simulink model "AUAV_V3_TestSensors"  (R2015a)
settings: Solver=FixedStepDiscrete  StartTime=0.0  StopTime=10.0  FixedStep=T  RelTol=1e-3
PreLoadFcn:
  | %T = 0.0025;
  | MavlinkBus;
  | mcuInit;
  | % Baro Altitude Computation
  | % =========================
  | basePressure = 98192.64;
  | baseTemp = 288.215;
  | lapseRate = -0.00198122;
  | baseHeight = 0;
values from neighbouring files (symbols this model uses):
  apSampleTime = 0.01    [mcuInit.m]
  latlong_WP = 1    [mcuInit.m]
  mavlink_attitude_t = Simulink.Bus    [MavlinkBusMarcello.m]
  mavlink_gps_raw_int_t = Simulink.Bus    [MavlinkBus.m]    (also in MavlinkBusMarcello.m)
  mavlink_raw_imu_t = Simulink.Bus    [MavlinkBus.m]    (also in MavlinkBusMarcello.m)
  mavlink_scaled_pressure_t = Simulink.Bus    [MavlinkBus.m]    (also in MavlinkBusMarcello.m)
  mavlink_servo_output_raw_t = Simulink.Bus    [MavlinkBusMarcello.m]
  mavlink_slugs_navigation_t = Simulink.Bus    [MavlinkBusMarcello.m]
  mavlink_sys_status_t = Simulink.Bus    [MavlinkBus.m]    (also in MavlinkBusMarcello.m)
  T = 0.01    [mcuInit.m]
  Xpoints = [0 0]    [mcuInit.m]
  Ypoints = [0 0]    [mcuInit.m]
  Zpoints = [0 0]    [mcuInit.m]
undefined symbols (not defined in the file or in its folder): A0, A14, A15, A2, A3, A4, A5, A6, accBiasRateLimit, B0, bankCommandLimit, barAdjust, baroCutoff, baroCutTemp, cubeAccelGain16405, cubeGyroGain16405, cubeMagGain16405, D0, D11, D7, D8, daLimit, data, daTrimMax, daTrimMin, deLimit, deTrimMax, deTrimMin, drLimit, drTrimMax, drTrimMin, dtLimit, dtTrimMax, dtTrimMin, F2, F3, G0, G13, G15, gaind, GS_location, gyroBiasRateLimit, IC1max, IPStar, ISA_g, Max, maxAcc, MaxDwnPthStar, maxDynPressure, maxEta, mlParamInterface, ms, OC1max, P112, P125, P127, P16, P20, P21, P30 ... (+26)
undefined symbols (not defined in the file): baroOffset, baroScale, barTGain1, barTGain2, barTMean1, barTMean2, bda, bde, bdr, bdt, bICda, bICde, bICdr, bICdt, derivativesConstant, lowRateSensorCutoff, mainSensorCutoff, mda, mde, mdr, mdt, mICda, mICde, mICdr, mICdt, pitotOffset, pitotScale, pitTGain1, pitTGain2, pitTMean1, pitTMean2, powerOffset, powerScale, pressureSensorCutoff, tempOffset, tempScale, vzCutoff, xCutoff, yCutoff
libraries: MCHP_Blockset x158, simulink x84, SLUGS_Library x31, aerolibconvert2 x6, aerolibutil x4, aerolibtransform2 x3, dspmtrx3 x2, aerolibobsolete x2
(part 9 of 24)

== system AUAV_V3_TestSensors/Inner Loop// Navigation/Longitudinal Channel Encaps [updated 4.28.16] ==
  U_c : Inport
  dyn P : Inport  Port=2
  U_hold PID Gains : Inport  Port=3
  dT_trim : Inport  Port=4
  h_c : Inport  Port=5
  h_m : Inport  Port=6
  he2th PI Gains : Inport  Port=7
  Roll to Height FF : Inport  Port=8
  theta_m : Inport  Port=9
  th2dE PID Gains : Inport  Port=10
  dE_trim : Inport  Port=11
  Manual? : Inport  Port=12
  phi_m : Inport  Port=13
  dt FF Gain : Inport  Port=14
  Constant3 : Constant  Value=[100 100 100]  OutDataTypeStr=single
  Longitudinal Channel : Subsystem  AncestorBlock=SLUGS_Library/Control Blocks/Longitudinal Channel
  mlNavigation : DataStoreWrite  DialogController=Simulink.DDGSource  DataStoreName=mlNavigation  DataStoreElements=mlNavigation.u_m#mlNavigation.theta_c#mlNavigation.h_c
  dE : Outport
  dT : Outport  Port=2
  theta_C : Outport  Port=3
  h_c_in : Outport  Port=4
  U_m : Outport  Port=5
  wires:
  U_c/1 -> Longitudinal Channel/1(U_c)
  dyn P/1 -> Longitudinal Channel/2(dyn P)
  U_hold PID Gains/1 -> Longitudinal Channel/3(U_hold PID Gains)
  dT_trim/1 -> Longitudinal Channel/4(dT_trim)
  h_m/1 -> Longitudinal Channel/6(h_m)
  theta_m/1 -> Longitudinal Channel/9(theta_m)
  dE_trim/1 -> Longitudinal Channel/11(dE_trim)
  Manual?/1 -> Longitudinal Channel/12(Manual?)
  he2th PI Gains/1 -> Longitudinal Channel/7(he2th PI Gains)
  Roll to Height FF/1 -> Longitudinal Channel/8(Roll to Height FF)
  th2dE PID Gains/1 -> Longitudinal Channel/10(th2dE PID Gains)
  dt FF Gain/1 -> Longitudinal Channel/14(dt FF Gain)
  h_c/1 -> Longitudinal Channel/5(h_c)
  phi_m/1 -> Longitudinal Channel/13(phi_m)
  Longitudinal Channel/1(dE) -> dE/1  "U"
  Longitudinal Channel/2(dT) -> dT/1
  Longitudinal Channel/3(h_c_in) -> mlNavigation/3, h_c_in/1
  Longitudinal Channel/4(U_m) -> mlNavigation/1, U_m/1
  Longitudinal Channel/5(theta_C) -> mlNavigation/2, theta_C/1
  Constant3/1 -> Longitudinal Channel/15(GS Location)

== system AUAV_V3_TestSensors/Inner Loop// Navigation/Navigation Encaps [updated 4.28.16] ==
  Puav : Inport  SampleTime=apSampleTime
  Max WP Idx : Inport  Port=2
  Vxyz : Inport  Port=3  SampleTime=apSampleTime
  T*(m) : Inport  Port=4
  U_c : Inport  Port=5
  WPFly : Inport  Port=6
  TurnLeadTime : Inport  Port=7
  RTB : Inport  Port=8
  Mobile Location : Inport  Port=9
  Follow Mobile? : Inport  Port=10
  MidLvl h_c : Inport  Port=11
  isApManual? : Inport  Port=12
  ISR Scale : Inport  Port=13
  Data Type Conversion : DataTypeConversion  OutDataTypeStr=uint8
  Get ISR Location : DataStoreRead  DialogController=Simulink.DDGSource  DataStoreName=mlISR  DataStoreElements=mlISR.latitude#mlISR.longitude#mlISR.height
  Get Nav Mode : DataStoreRead  DialogController=Simulink.DDGSource  DataStoreName=mlHeartbeatLocal  DataStoreElements=mlHeartbeatLocal.custom_mode
  Mux : Mux  Inputs=3
  Navigation : Subsystem  AncestorBlock=SLUGS_Library/Navigation/Navigation
  h_c : Outport
  phi_c : Outport  Port=2
  ISR Loc : Outport  Port=3
  "Puav " : Outport  Port=4
  wires:
  T*(m)/1 -> Navigation/2(T*(m))
  WPFly/1 -> Navigation/3(WPFly)
  RTB/1 -> Navigation/4(RTB)
  isApManual?/1 -> Navigation/5(isApManual?)
  Navigation/1(h_c) -> h_c/1
  Navigation/2(phi_c) -> phi_c/1
  Puav/1 -> Navigation/6(Puav)
  Navigation/4("Puav ") -> "Puav "/1
  Max WP Idx/1 -> Navigation/8(Max WP Idx)
  Vxyz/1 -> Navigation/9(Vxyz)
  U_c/1 -> Navigation/10(U_c)
  TurnLeadTime/1 -> Navigation/11(TurnLeadTime)
  Mobile Location/1 -> Navigation/12(Mobile Location)
  Follow Mobile?/1 -> Navigation/13(Follow Mobile?)
  MidLvl h_c/1 -> Navigation/14(MidLvl h_c)
  ISR Scale/1 -> Navigation/15(ISR Scale)
  Navigation/3(ISR Loc) -> ISR Loc/1
  Mux/1 -> Navigation/7(ISR Location)
  Get ISR Location/2 -> Mux/2
  Get ISR Location/1 -> Mux/1
  Get ISR Location/3 -> Mux/3
  Get Nav Mode/1 -> Data Type Conversion/1
  Data Type Conversion/1 -> Navigation/1(NavMode)

== system AUAV_V3_TestSensors/Inner Loop// Navigation/Protect NaNs ==
  In1 : Inport
  Integer Delay3 : Delay  DelayLength=1  InputProcessing=Inherited  SampleTime=T
  Relational Operator2 : RelationalOperator  Operator===  OutDataTypeStr=uint(8)
  Switch3 : Switch  Criteria=u2 > Threshold  Threshold=0.3  SampleTime=.01
  Out1 : Outport
  wires:
  Integer Delay3/1 -> Switch3/3
  Switch3/1 -> Out1/1, Integer Delay3/1
  In1/1 -> Relational Operator2/2, Relational Operator2/1, Switch3/1
  Relational Operator2/1 -> Switch3/2

== system AUAV_V3_TestSensors/Position_and_Attitude_Filter/Attitude Complimentary Filter COG ==
  A_sens : Inport  PortDimensions=3
  XY Orient : Inport  Port=2  OutDataTypeStr=single
  Gyros : Inport  Port=3  PortDimensions=3
  Vxyd_hat : Inport  Port=4  PortDimensions=3
  acc_bias : Inport  Port=5  PortDimensions=3
  3D Filter : Subsystem  AncestorBlock=SLUGS_Library/Singnal Routing & Conditioning/3D Filter  RTWFcnName=TustinFilter3D  mask{zval=[], pval=[0], kval=1, TSample=0.01}
      mask prompts: zval "Zeros"; pval "Poles"; kval "Gains"; TSample "Sample Time"
      settings: RTWFcnNameOpts=User specified  RTWFileNameOpts=Use function name
      mask Display:
      | droots(zval,pval,kval)
      | port_label('input',1,'3D')
  3x3 Cross Product : aerolibutil/3x3 Cross Product
  3x3 Cross Product1 : aerolibutil/3x3 Cross Product
  3x3 Cross Product2 : aerolibutil/3x3 Cross Product
  Add : Sum  Inputs=++--
  Bias Rate Limiter : RateLimiter  RisingSlewLimit=gyroBiasRateLimit  FallingSlewLimit=-gyroBiasRateLimit  SampleTimeMode=inherited
  Constant1 : Constant  Value=0  OutDataTypeStr=single
  Data Type Conversion : DataTypeConversion  OutDataTypeStr=single
  Demux : Demux  Outputs=3
  Demux1 : Demux  Outputs=3
  "Deriv " : Subsystem
  Direction Cosine Matrix to Rotation Angles : aerolibtransform2/Direction Cosine Matrix to Rotation Angles  rotationOrder=ZYX  lim=Default
      settings: AttributesFormatString=Rotation Order: %<rotationOrder>
  Discrete-Time Integrator1 : DiscreteIntegrator  InitialCondition=q_quat  SampleTime=apSampleTime  LimitOutput=on  UpperSaturationLimit=[1 1 1 1]  LowerSaturationLimit=[-1 -1 -1 -1]
  Embedded MATLAB Function : MATLAB Function  TreatAsAtomicUnit=on
  Gain : Gain  Gain=0.1
  Gain1 : Gain  Gain=30
  Integer Delay : Delay  DelayLength=1  InputProcessing=Inherited
  Mux : Mux  Inputs=3
  Normalize Vector1 : Subsystem  AncestorBlock=SLUGS_Library/Navigation/Normalize Vector
  Normalize Vector2 : Subsystem  AncestorBlock=SLUGS_Library/Navigation/Normalize Vector
  Product1 : Product  Multiplication=Matrix(*)  RndMeth=Zero
  Product2 : Product  Multiplication=Matrix(*)  RndMeth=Zero
  Quaternion Normalize : aerolibutil/Quaternion Normalize
  Quaternions to Direction Cosine Matrix : aerolibtransform2/Quaternions to  Direction Cosine Matrix
  Submatrix : dspmtrx3/Submatrix  RowSpan=Range of rows  RowStartMode=First  RowStartIndex=1  RowEndMode=Last  RowEndIndex=1  ColSpan=One column  ColStartMode=Last  ColStartIndex=1  ColEndMode=Last  ColEndIndex=1
  Submatrix1 : dspmtrx3/Submatrix  RowSpan=One row  RowStartMode=First  RowStartIndex=1  RowEndMode=Last  RowEndIndex=1  ColSpan=All columns  ColStartMode=Last  ColStartIndex=1  ColEndMode=Last  ColEndIndex=1
  Sum1 : Sum  Inputs=++|
  Sum3 : Sum  Inputs=++|
  Sum4 : Sum  Inputs=++|
  myMux Fun2 : MATLAB Function  TreatAsAtomicUnit=on
  q dot calc : MATLAB Function  TreatAsAtomicUnit=on
  euler_hat : Outport
  pqr_hat : Outport  Port=2
  Gyro Bias : Outport  Port=3
  RL2B : Outport  Port=4
  wires:
  Bias Rate Limiter/1 -> Gyro Bias/1, Sum3/2
  Product2/1 -> Gain1/1
  Gain1/1 -> Sum4/1
  Normalize Vector2/1(Normalized) -> 3x3 Cross Product2/1
  myMux Fun2/1(y) -> Normalize Vector2/1(Vector)
  Constant1/1 -> myMux Fun2/3(u3)
  Demux1/2 -> myMux Fun2/2(u2)
  Demux1/1 -> myMux Fun2/1(u1)
  Submatrix1/1 -> Demux1/1
  Sum1/1 -> q dot calc/2(om_hat), Integer Delay/1  "om_hat"
  q dot calc/1(q_dot) -> Discrete-Time Integrator1/1
  Submatrix/1 -> 3x3 Cross Product/2  "g_hat"
  Sum4/1 -> Gain/1, 3D Filter/1(In1)
  3x3 Cross Product1/1 -> Add/1
  A_sens/1 -> Add/3
  Normalize Vector1/1(Normalized) -> 3x3 Cross Product/1
  3x3 Cross Product/1 -> Sum4/2
  Quaternions to Direction Cosine Matrix/1 -> Submatrix1/1, Product2/1, Product1/1, Submatrix/1, RL2B/1, Direction Cosine Matrix to Rotation Angles/1  "RLT2B"
  Integer Delay/1 -> 3x3 Cross Product1/1
  Discrete-Time Integrator1/1 -> Quaternion Normalize/1  "q1"
  Quaternion Normalize/1 -> Quaternions to Direction Cosine Matrix/1, q dot calc/1(q)
  "Deriv "/1(ydot) -> Add/2
  Add/1 -> Normalize Vector1/1(Vector)
  acc_bias/1 -> Add/4
  Product1/1 -> 3x3 Cross Product1/2, "Deriv "/1(y)
  Vxyd_hat/1 -> Product1/2
  3D Filter/1(Out1) -> Bias Rate Limiter/1
  Gyros/1 -> Sum3/1
  Gain/1 -> Sum1/2
  Sum3/1 -> Sum1/1, pqr_hat/1  "Gyro Err"
  XY Orient/1 -> 3x3 Cross Product2/2
  3x3 Cross Product2/1 -> Product2/2
  Demux/1 -> Embedded MATLAB Function/1(u)
  Mux/1 -> euler_hat/1
  Embedded MATLAB Function/1(y) -> Mux/3
  Direction Cosine Matrix to Rotation Angles/1 -> Data Type Conversion/1
  Demux/2 -> Mux/2
  Demux/3 -> Mux/1
  Data Type Conversion/1 -> Demux/1

== system AUAV_V3_TestSensors/Position_and_Attitude_Filter/COG.SOG2V ==
  COG_D : Inport
  SOG : Inport  Port=2
  Angle Conversion : aerolibconvert2/Angle Conversion  IU=deg  OU=rad
  Constant : Constant  Value=0  OutDataTypeStr=single
  Product : Product  RndMeth=Zero
  Product1 : Product  RndMeth=Zero
  Subsystem5 : Subsystem  AncestorBlock=SLUGS_Library/Subsystem5
  myMux Fun2 : MATLAB Function  TreatAsAtomicUnit=on
  Vnorth : Outport
  Veast : Outport  Port=2
  XY Orient : Outport  Port=3
  wires:
  Product1/1 -> Vnorth/1
  Product/1 -> Veast/1
  SOG/1 -> Product1/1, Product/2
  Angle Conversion/1 -> Subsystem5/1(u)
  Subsystem5/1(sin(u)) -> Product/1, myMux Fun2/2(u2)
  Subsystem5/2(cos(u)) -> Product1/2, myMux Fun2/1(u1)
  COG_D/1 -> Angle Conversion/1
  Constant/1 -> myMux Fun2/3(u3)
  myMux Fun2/1(y) -> XY Orient/1

== system AUAV_V3_TestSensors/Position_and_Attitude_Filter/Compute GS Location ==
  GS Location : Inport
  Demux : Demux  Outputs=3
  Geod2ECEF1 : Subsystem  mask{Re=6378137, Rp=6356752.3142}
      mask prompts: Re "Enter equatorial radius, m"; Rp "Enter polar radius,m"
  Mux1 : Mux  Inputs=2
  Mux2 : Mux  Inputs=3
  "Lat, Lon" : Outport
  R_in : Outport  Port=2
  wires:
  Geod2ECEF1/3("Ze, m ") -> Mux2/3
  Geod2ECEF1/1("Xe, m ") -> Mux2/1
  Geod2ECEF1/2("Ye, m ") -> Mux2/2
  Demux/1 -> Geod2ECEF1/1("height, m")
  Demux/2 -> Mux1/2, Geod2ECEF1/2("lat, deg")
  Demux/3 -> Mux1/1, Geod2ECEF1/3(lon,deg)
  GS Location/1 -> Demux/1
  Mux1/1 -> "Lat, Lon"/1
  Mux2/1 -> R_in/1  "R_in"

== system AUAV_V3_TestSensors/Position_and_Attitude_Filter/Enabled Subsystem ==
  In1 : Inport
  In2 : Inport  Port=2
  In3 : Inport  Port=3
  Enable : EnablePort
  Out1 : Outport
  Out2 : Outport  Port=2
  Out3 : Outport  Port=3
  wires:
  In1/1 -> Out1/1
  In2/1 -> Out2/1
  In3/1 -> Out3/1

== system AUAV_V3_TestSensors/Position_and_Attitude_Filter/GPS Update ==
  XYZ : Inport
  Data Type Conversion2 : DataTypeConversion  OutDataTypeStr=uint8
  Demux : Demux  Outputs=3
  Detect Change : Subsystem
  Detect Change1 : Subsystem
  Detect Change2 : Subsystem
  Rate Transition : RateTransition  OutPortSampleTime=T
  Saturation1 : Saturate  UpperLimit=1  LowerLimit=0  SampleTime=T
  Sum : Sum  Inputs=3
  Update? : Outport
  wires:
  Demux/1 -> Detect Change/1(Data)
  Demux/2 -> Detect Change1/1(Data)
  Demux/3 -> Detect Change2/1(Data)
  Detect Change/1(change?) -> Sum/1
  Detect Change1/1(change?) -> Sum/2
  Detect Change2/1(change?) -> Sum/3
  Sum/1 -> Saturation1/1
  XYZ/1 -> Rate Transition/1
  Saturation1/1 -> Data Type Conversion2/1
  Rate Transition/1 -> Demux/1
  Data Type Conversion2/1 -> Update?/1

== system AUAV_V3_TestSensors/Position_and_Attitude_Filter/Geod2LTP1 ==
  GS Lat,Lon : Inport
  GS ECEF : Inport  Port=2
  "Lat, deg(GPS)" : Inport  Port=3
  "Lon, deg(GPS)" : Inport  Port=4
  Hight,m(GPS) : Inport  Port=5
  ECEF2LTP (UEN) : Subsystem
      mask Display: plot(0,0,100,100,[45,40,35,40,40],[85,95,85,95,40],[85,95,85,95,40],[35,40,45,40,40],[60,40,10,20,10,14],[70,40,10,13,10,20],[56,45],[70,70],[60,60],[50,60],[60,60],[30,40],[50,60],[20,20],[30,40],[20,20],[45,55],[35,25],[75,65],[35,25])
  Geod2ECEF1 : Subsystem  mask{Re=6378137, Rp=6356752.3142}
      mask prompts: Re "Enter equatorial radius, m"; Rp "Enter polar radius,m"
  Mux : Mux  Inputs=3
  Reshape : Reshape  OutputDimensionality=Column vector (2-D)
  Reshape1 : Reshape
  Sum1 : Sum  Inputs=|+-  OutDataTypeStr=single  SaturateOnIntegerOverflow=on
  UEN 2 NEU : Gain  Gain=[0 0 1;0 1 0;1 0 0]  Multiplication=Matrix(K*u)  OutDataTypeStr=float('single')  SaturateOnIntegerOverflow=on  ParamDataTypeStr=Inherit: Same as input
  "NEU, m" : Outport
  wires:
  Reshape1/1 -> "NEU, m"/1
  Reshape/1 -> UEN 2 NEU/1
  Sum1/1 -> ECEF2LTP (UEN)/1(ECEF coordinates)
  Mux/1 -> Sum1/1  "r_mov"
  Hight,m(GPS)/1 -> Geod2ECEF1/1("height, m")
  ECEF2LTP (UEN)/1(Out) -> Reshape/1  "Moving Side"
  GS ECEF/1 -> Sum1/2
  GS Lat,Lon/1 -> ECEF2LTP (UEN)/2("Long, Lat")
  "Lon, deg(GPS)"/1 -> Geod2ECEF1/3(lon,deg)
  "Lat, deg(GPS)"/1 -> Geod2ECEF1/2("lat, deg")
  Geod2ECEF1/2("Ye, m ") -> Mux/2
  Geod2ECEF1/1("Xe, m ") -> Mux/1
  Geod2ECEF1/3("Ze, m ") -> Mux/3
  UEN 2 NEU/1 -> Reshape1/1

== system AUAV_V3_TestSensors/Position_and_Attitude_Filter/Position Filter ==
  NewGPS : Inport
  Baro Alt : Inport  Port=2
  RLT2B : Inport  Port=3
  GPS_XYD : Inport  Port=4
  Vnorth : Inport  Port=5
  Veast : Inport  Port=6
  SOG : Inport  Port=7
  A_sens(m/s^2) : Inport  Port=8
  Base Height (m) : Inport  Port=9
  BlendPosVel : Subsystem
  Vxyd_hat : Outport
  Pxyd_hat : Outport  Port=2
  acc_bias : Outport  Port=3
  wires:
  BlendPosVel/3(acc_bias) -> acc_bias/1
  BlendPosVel/1(Vxyd_hat) -> Vxyd_hat/1
  BlendPosVel/2(Pxyd_hat) -> Pxyd_hat/1
  Baro Alt/1 -> BlendPosVel/4(BaroAlt)
  Veast/1 -> BlendPosVel/3(Veast)
  Vnorth/1 -> BlendPosVel/2(Vnorth)
  NewGPS/1 -> BlendPosVel/6(NewGPS)
  RLT2B/1 -> BlendPosVel/5(RLT2B)
  GPS_XYD/1 -> BlendPosVel/1(GPS_NED)
  SOG/1 -> BlendPosVel/7(SOG)
  A_sens(m/s^2)/1 -> BlendPosVel/8(A_sens(m/s^2))
  Base Height (m)/1 -> BlendPosVel/9(Base Height)

== system AUAV_V3_TestSensors/RC_Driver/Mixing ==
  note: Pitch positif : go down
      | Yaw positive : turn left
  Pitch : Inport
  Roll : Inport  Port=2
  Sum : Sum  Inputs=-+  SaturateOnIntegerOverflow=on  OutDataTypeStr=Inherit: Same as first input
  Sum1 : Sum  SaturateOnIntegerOverflow=on  OutDataTypeStr=Inherit: Same as first input
  Cmd Servo Left : Outport
  Cmd Servo Right : Outport  Port=2
  wires:
  Pitch/1 -> Sum1/1, Sum/1
  Roll/1 -> Sum/2, Sum1/2
  Sum/1 -> Cmd Servo Left/1
  Sum1/1 -> Cmd Servo Right/1

== system AUAV_V3_TestSensors/Sensor_Data_Adapter/Initialize GS Location ==
  Enable : EnablePort
  Constant : Constant  Value=0
  Data Store Read1 : DataStoreRead  DataStoreName=mlGpsData  DataStoreElements=mlGpsData.lat#mlGpsData.lon#mlGpsData.alt
  Data Store Write : DataStoreWrite  DataStoreName=GS_INIT_FLAG
  Data Store Write1 : DataStoreWrite  DialogController=Simulink.DDGSource  DataStoreName=mlGSLocationFloat  DataStoreElements=mlGSLocationFloat.lat#mlGSLocationFloat.lon#mlGSLocationFloat.alt
  Data Type Conversion : DataTypeConversion
  Data Type Conversion1 : DataTypeConversion
  Data Type Conversion2 : DataTypeConversion
  wires:
  Data Store Read1/1 -> Data Type Conversion/1
  Data Store Read1/2 -> Data Type Conversion1/1
  Constant/1 -> Data Store Write/1
  Data Store Read1/3 -> Data Type Conversion2/1
  Data Type Conversion/1 -> Data Store Write1/1
  Data Type Conversion1/1 -> Data Store Write1/2
  Data Type Conversion2/1 -> Data Store Write1/3

== system AUAV_V3_TestSensors/Sensor_Data_Adapter/Raw HIL Readings ==
  Enable : EnablePort
  Data Store Read : DataStoreRead  DataStoreName=SIX_DOF_HIL_FLAG
  Data Store Read1 : DataStoreRead  DataStoreName=X_PLANE_HIL_FLAG
  Enabled Subsystem : Subsystem  TreatAsAtomicUnit=on
  Enabled Subsystem1 : Subsystem  TreatAsAtomicUnit=on
  MATLAB Function : MATLAB Function  Commented=on  TreatAsAtomicUnit=on
  Switch : Switch  Criteria=u2 ~= 0  SampleTime=0.01
  Raw Msg : Outport
  wires:
  Switch/1 -> Raw Msg/1
  Data Store Read/1 -> Enabled Subsystem/Enable
  Data Store Read1/1 -> Switch/2, Enabled Subsystem1/Enable
  Enabled Subsystem1/1(Out2) -> Switch/1
  Enabled Subsystem/1(Out2) -> Switch/3

== system AUAV_V3_TestSensors/Sensor_Data_Adapter/Sensor Suite ==
  HIL_flag : Inport
  Raw HIL : Inport  Port=2
  " GPS is Ublox" : Subsystem
  "ADIS16405 Signal Cond " : Subsystem
  Compute CPU Load : Subsystem
  Constant : Constant
  Data Type Conversion{4..7} (4 alike) : DataTypeConversion  OutDataTypeStr=single
  Demux : Demux
  Demux1 : Demux
  Goto4 : Goto  Commented=on  GotoTag=IntDiag
  Goto5 : Goto  Commented=on  GotoTag=charDiag
  If no HIL then Read all the Sensors : Subsystem
  If no HIL then update Air Data : Subsystem
  Logical Operator : Logic  Operator=NOT  AllPortsSameDT=off  OutDataTypeStr=boolean
  Low Pass Filtering,Temperature Compensation and Calibration : Subsystem
  Sensor DSC Diag [updateSensorMcuState.c]1 : MCHP_Blockset/User Functions/C Function Call  ParseFilesChkbx=off  ListFunctions1=Custom Function  Function1=extern void updateSensorDiag(real32_T* u1);  AddHeaderDeclaration=on  Function1Type=when block is updated (default)  Fct1BlockIn=u1[4]  FctReturnBlockOut=off  DataCollected=0  ORDERING=None  SampleTime=.01  MCHP_MASTERLINK=|  PinDigitalInput=[]  PinDigitalOutput=[]  PinAnalogInput=[]
      | AUAV_V3_TestSensors/Microchip Master
      | AUAV V3 Board
      | Busy Flag on D2 (RA6)
  Switch : Switch  Criteria=u2 ~= 0  SampleTime=0.01
  Switch1 : Switch  Criteria=u2 ~= 0  SampleTime=0.01
  Update the Load and Power Data [updateSensorMcuState.c]1 : MCHP_Blockset/User Functions/C Function Call  ParseFilesChkbx=off  ListFunctions1=Custom Function  Function1=extern void updateLoadData(uint8_T u1, uint16_T u2);  AddHeaderDeclaration=on  Function1Type=when block is updated (default)  FctReturnBlockOut=off  DataCollected=0  ORDERING=None  SampleTime=.01  MCHP_MASTERLINK=|  PinDigitalInput=[]  PinDigitalOutput=[]  PinAnalogInput=[]
      | AUAV_V3_TestSensors/Microchip Master
      | AUAV V3 Board
      | Busy Flag on D2 (RA6)
  myMux Fun : MATLAB Function  TreatAsAtomicUnit=on
  myMux Fun1 : MATLAB Function  TreatAsAtomicUnit=on
  Omega (rad/s) : Outport
  Accel (m/s^2) : Outport  Port=2
  Mag (mG) : Outport  Port=3
  Baro Alt (m) : Outport  Port=4
  GPS : Outport  Port=5
  wires:
  If no HIL then Read all the Sensors/1(Sensors) -> Switch/3
  Logical Operator/1 -> If no HIL then Read all the Sensors/Enable, [Not_HIL]
  Demux/1 -> "ADIS16405 Signal Cond "/1(Gyro Raw)  "Gyro"
  Demux1/1 -> Low Pass Filtering,Temperature Compensation and Calibration/1(Baro raw)
  Demux1/2 -> Low Pass Filtering,Temperature Compensation and Calibration/2(Pitot raw)
  Demux1/4 -> Low Pass Filtering,Temperature Compensation and Calibration/4(Therm Raw)
  Demux/3 -> "ADIS16405 Signal Cond "/3(Mag Raw)  "Mag"
  Demux1/3 -> Low Pass Filtering,Temperature Compensation and Calibration/3(Power Raw)
  Low Pass Filtering,Temperature Compensation and Calibration/2(Pitot (Pa)) -> myMux Fun/1(u1), [Float1Diag]
  Low Pass Filtering,Temperature Compensation and Calibration/3(Static (Pa)) -> myMux Fun/2(u2)
  myMux Fun/1(y) -> If no HIL then update Air Data/1(AirData)
  Low Pass Filtering,Temperature Compensation and Calibration/4(Temp (0.1 C)) -> myMux Fun/3(u3)
  Compute CPU Load/1(Load (%)) -> Update the Load and Power Data [updateSensorMcuState.c]1/1
  Low Pass Filtering,Temperature Compensation and Calibration/5(Power (V)) -> Update the Load and Power Data [updateSensorMcuState.c]1/2
  Demux/2 -> "ADIS16405 Signal Cond "/2(Accel Raw)  "Accel"
  myMux Fun1/1(y) -> Sensor DSC Diag [updateSensorMcuState.c]1/1
  Data Type Conversion5/1 -> myMux Fun1/1(u1)  "float"
  Data Type Conversion4/1 -> myMux Fun1/2(u2)  "float"
  Data Type Conversion6/1 -> myMux Fun1/3(u3)  "int"
  Data Type Conversion7/1 -> myMux Fun1/4(u4)  "char"
  [Float1Diag] -> Data Type Conversion5/1
  [Float2Diag] -> Data Type Conversion4/1
  [IntDiag] -> Data Type Conversion6/1
  [charDiag] -> Data Type Conversion7/1
  If no HIL then update Air Data/1(Out1) -> [Float2Diag]
  "ADIS16405 Signal Cond "/1(Omega (rad/s)) -> Omega (rad/s)/1
  "ADIS16405 Signal Cond "/2(Accel (m/s^2)) -> Accel (m/s^2)/1
  "ADIS16405 Signal Cond "/3(Mags (mG)) -> Mag (mG)/1
  Raw HIL/1 -> Switch/1
  HIL_flag/1 -> [HIL], Switch/2, Logical Operator/1
  Switch/1 -> Demux/1
  Low Pass Filtering,Temperature Compensation and Calibration/1(Baro Alt (m)) -> Baro Alt (m)/1
  Demux/4 -> Demux1/1
  [Not_HIL] -> Switch1/2
  Switch1/1 -> GPS/1
  " GPS is Ublox"/1(GPS Main) -> Switch1/3
  If no HIL then Read all the Sensors/2(GPS) -> Switch1/1
  Constant/1 -> If no HIL then update Air Data/Enable

== system AUAV_V3_TestSensors/Servo In Out/Convert to Microseconds ==
  PWM : Inport
  Convert to Microseconds : Gain  Gain=0.4
  Data Type Conversion : DataTypeConversion  OutDataTypeStr=uint16
  uS : Outport
  wires:
  Data Type Conversion/1 -> uS/1
  PWM/1 -> Convert to Microseconds/1
  Convert to Microseconds/1 -> Data Type Conversion/1

== system AUAV_V3_TestSensors/Servo In Out/Convert to Microseconds1 ==
  PWM : Inport
  Convert to Microseconds : Gain  Gain=0.4
  Data Type Conversion : DataTypeConversion  OutDataTypeStr=uint16
  uS : Outport
  wires:
  Data Type Conversion/1 -> uS/1
  PWM/1 -> Convert to Microseconds/1
  Convert to Microseconds/1 -> Data Type Conversion/1

== system AUAV_V3_TestSensors/Servo In Out/Convert to Microseconds2 ==
  PWM : Inport
  Convert to Microseconds : Gain  Gain=0.4
  Data Type Conversion : DataTypeConversion  OutDataTypeStr=uint16
  uS : Outport
  wires:
  Data Type Conversion/1 -> uS/1
  PWM/1 -> Convert to Microseconds/1
  Convert to Microseconds/1 -> Data Type Conversion/1

== system AUAV_V3_TestSensors/Servo In Out/Mixing ==
  note: Pitch positif : go down
      | Yaw positive : turn left
  Pitch : Inport
  Roll : Inport  Port=2
  Sum : Sum  Inputs=-+  SaturateOnIntegerOverflow=on  OutDataTypeStr=Inherit: Same as first input
  Sum1 : Sum  SaturateOnIntegerOverflow=on  OutDataTypeStr=Inherit: Same as first input
  Cmd Servo Left : Outport
  Cmd Servo Right : Outport  Port=2
  wires:
  Pitch/1 -> Sum1/1, Sum/1
  Roll/1 -> Sum/2, Sum1/2
  Sum/1 -> Cmd Servo Left/1
  Sum1/1 -> Cmd Servo Right/1

== system AUAV_V3_TestSensors/Trim Vals [updated 4.28.16]/Bufffer IC ==
  Pilot Console : Inport
  Buffer IC Channel : MATLAB Function  TreatAsAtomicUnit=on
  Buffer IC Channel1 : MATLAB Function  TreatAsAtomicUnit=on
  Buffer IC Channel2 : MATLAB Function  TreatAsAtomicUnit=on
  Buffer IC Channel3 : MATLAB Function  TreatAsAtomicUnit=on
  Demux : Demux
  dT_buf : Outport
  dA_buf : Outport  Port=2
  dR_buf : Outport  Port=3
  dE_buf : Outport  Port=4
  wires:
  Demux/1 -> Buffer IC Channel/1(latest)
  Demux/2 -> Buffer IC Channel1/1(latest)
  Demux/3 -> Buffer IC Channel2/1(latest)
  Demux/4 -> Buffer IC Channel3/1(latest)
  Pilot Console/1 -> Demux/1
  Buffer IC Channel/1(history) -> dT_buf/1
  Buffer IC Channel1/1(history) -> dA_buf/1
  Buffer IC Channel2/1(history) -> dR_buf/1
  Buffer IC Channel3/1(history) -> dE_buf/1

== system AUAV_V3_TestSensors/Trim Vals [updated 4.28.16]/Control Surface Input ==
  2 sec  tau : Subsystem  mask(Tustin1stOrderLowpassAutoInitialCondition){f=0.1, T=T}
      mask prompts: f "Lowpass Frequency"; T "Sample Time"
      mask help: Takes a 3db rolloff frequency (in Hz, NOT radians/s) and a sample time. Performs a symbolic Tustin conversion and implements in a discrete filter. The initial output of the filter is set by the first sample.
      mask Help: Enter the desired 3db rolloff frequency in Hz and the sample time. Initial conditions are sampled automatically.
      mask Display: fprintf('%.2f Hz lowpass',f)
  2 sec  tau1 : Subsystem  mask(Tustin1stOrderLowpassAutoInitialCondition){f=0.1, T=T}
      mask prompts: f "Lowpass Frequency"; T "Sample Time"
      mask help: Takes a 3db rolloff frequency (in Hz, NOT radians/s) and a sample time. Performs a symbolic Tustin conversion and implements in a discrete filter. The initial output of the filter is set by the first sample.
      mask Help: Enter the desired 3db rolloff frequency in Hz and the sample time. Initial conditions are sampled automatically.
      mask Display: fprintf('%.2f Hz lowpass',f)
  Data Type Conversion1 : DataTypeConversion  OutDataTypeStr=uint16
  Data Type Conversion2 : DataTypeConversion  OutDataTypeStr=single
  Data Type Conversion3 : DataTypeConversion  OutDataTypeStr=single
  Data Type Conversion4 : DataTypeConversion  OutDataTypeStr=uint16
  Input Capture : MCHP_Blockset/Pulse Input//Output/Input Capture  IntPriority=6  Channel="[1     2     3     4     5     6     7     8]"  Channel_OLD="[1  2  3  4  5  6  7  8]"  PIN_IC1=Dynamic Options  PIN_IC1_TXT=D0 / P64 / Pin[72]  PIN_IC2=Dynamic Options  PIN_IC2_TXT=D8 / P72 / Pin[68]  PIN_IC3=Dynamic Options  PIN_IC3_TXT=D11 / P75 / Pin[71]  PIN_IC4=Dynamic Options  PIN_IC4_TXT=A15 / P31 / Pin[67]  PIN_IC5=Dynamic Options  PIN_IC5_TXT=A5 / P21 / Pin[61]  PIN_IC6=Dynamic Options  PIN_IC6_TXT=A14 / P30 / Pin[66]  PIN_IC7=Dynamic Options  PIN_IC7_TXT=A4 / P20 / Pin[60]  PIN_IC8=Dynamic Options  PIN_IC8_TXT=A0 / P16 / Pin[17]  PIN_IC9=Dynamic Options  PIN_IC9_TXT=A0 / P16 / Pin[17]  PIN_IC10=Dynamic Options  PIN_IC10_TXT=A0 / P16 / Pin[17]  PIN_IC11=Dynamic Options  PIN_IC11_TXT=A0 / P16 / Pin[17]  PIN_IC12=Dynamic Options  PIN_IC12_TXT=A0 / P16 / Pin[17]  PIN_IC13=Dynamic Options  PIN_IC13_TXT=A0 / P16 / Pin[17]  PIN_IC14=Dynamic Options  PIN_IC14_TXT=A0 / P16 / Pin[17]  PIN_IC15=Dynamic Options  PIN_IC15_TXT=A0 / P16 / Pin[17]  PIN_IC16=Dynamic Options  PIN_IC16_TXT=A0 / P16 / Pin[17]  Channel_UP_Down_Periode="[1     1     1     1     1     1     1     1]"  MaxChannel="[0.003   0.003   0.003   0.003   0.003   0.003   0.003   0.003]"  SafeMarge="[0     0     0     0     0     0     0     0]"  MaxChannelValue="2.^[ 14.680  14.680  14.680  14.680  14.680  14.680  14.680  14.680]  =>  [26249  26249  26249  26249  26249  26249  26249  26249]"  ICxmax="[26249  26249  26249  26249  26249  26249  26249  26249]"  Timer="[1  1  1  1  1  1  1  1]"  ChangeDetected="[0     0     0     0     0     0     0     0]"  ChangeDetectedPortRef=3  SampleTime=.01  Status=OK  MCHP_PORT={Input Capture 1}{IC1}6:0:P64;{Input Capture 2}{IC2}6:0:P72;{Input Capture 3}{IC3}6:0:P75;{Input Capture 4}{IC4}6:0:P31;{Input Capture 5}{IC5}6:0:P21;{Input Capture 6}{IC6}6:0:P30;{Input Capture 7}{IC7}6:0:P20;{Input Capture 8}{IC8}6:0:P16;  MCHP_TIMER_REQUEST="{Input Capture 1}{IC1}6:0:1:0:[1  2  3  4  5]:210000;{Input Capture 1}{IC1}6:0:1:0:[1  2  3  4  5]:210000;{Input Capture 1}{IC1}6:0:1:0:[1  2  3  4  5]:210000;{Input Capture 1}{IC1}6:0:1:0:[1  2  3  4  5]:210000;{Input Capture 1}{IC1}6:0:1:0:[1  2  3  4  5]:210000;{Input Capture 1}{IC1}6:0:1:0:[1  2  3  4  5]:210000;{Input Capture 1}{IC1}6:0:1:0:[1  2  3  4  5]:210000;{Input Capture 1}{IC1}6:0:1:0:[1  2  3  4  5]:210000;"  MCHP_TIMER_RESULT=[1 26249.000000000011 ;1 26249.000000000011 ;1 26249.000000000011 ;1 26249.000000000011 ;1 26249.000000000011 ;1 26249.000000000011 ;1 26249.000000000011 ;1 26249.000000000011 ]  MCHP_MASTERLINK=|
      | AUAV_V3_TestSensors/Microchip Master
      | AUAV V3 Board
      | Busy Flag on D2 (RA6)
  Update Control Surface DATA : DataStoreWrite  DialogController=Simulink.DDGSource  DataStoreName=mlPilotConsoleData  DataStoreElements=mlPilotConsoleData.chan1_raw#mlPilotConsoleData.chan2_raw#mlPilotConsoleData.chan3_raw#mlPilotConsoleData.chan4_raw#mlPilotConsoleData.chan5_raw#mlPilotConsoleData.chan6_raw#mlPilotConsoleData.chan7_raw#mlPilotConsoleData.chan8_raw
  myMux Fun1 : MATLAB Function  TreatAsAtomicUnit=on
  myMux Fun5 : MATLAB Function  TreatAsAtomicUnit=on
  Pilot Console : Outport
  Voltage/Current Sensor : Outport  Port=2
  wires:
  Input Capture/7 -> Data Type Conversion3/1, Update Control Surface DATA/7
  myMux Fun1/1(y) -> Voltage/Current Sensor/1
  Input Capture/6 -> Update Control Surface DATA/6, Data Type Conversion2/1
  2 sec  tau/1(Out1) -> Data Type Conversion1/1
  2 sec  tau1/1(Out1) -> Data Type Conversion4/1
  Data Type Conversion1/1 -> myMux Fun1/1(u1)
  Data Type Conversion4/1 -> myMux Fun1/2(u2)
  Data Type Conversion2/1 -> 2 sec  tau/1(In1)
  Data Type Conversion3/1 -> 2 sec  tau1/1(In1)
  Input Capture/1 -> myMux Fun5/1(u1), Update Control Surface DATA/1
  Input Capture/4 -> myMux Fun5/4(u4), Update Control Surface DATA/4
  Input Capture/5 -> myMux Fun5/5(u5), Update Control Surface DATA/5
  Input Capture/2 -> myMux Fun5/2(u2), Update Control Surface DATA/2
  Input Capture/3 -> myMux Fun5/3(u3), Update Control Surface DATA/3
  myMux Fun5/1(y) -> Pilot Console/1
  Input Capture/8 -> Update Control Surface DATA/8

== system AUAV_V3_TestSensors/Trim Vals [updated 4.28.16]/Convert to Microseconds  ==
  IC : Inport
  Convert to Microseconds : Gain  Gain=0.2
  Data Type Conversion : DataTypeConversion  OutDataTypeStr=uint16
  uS : Outport
  wires:
  Convert to Microseconds/1 -> Data Type Conversion/1
  IC/1 -> Convert to Microseconds/1
  Data Type Conversion/1 -> uS/1

== system AUAV_V3_TestSensors/Trim Vals [updated 4.28.16]/Detect Transition High to Low ==
  Switch : Inport
  IC1 : InitialCondition  Value=0
  Logical Operator : Logic  Operator=NOT  AllPortsSameDT=off  OutDataTypeStr=boolean
  Subsystem : Subsystem
  Transition : Outport
  wires:
  Switch/1 -> Logical Operator/1
  IC1/1 -> Subsystem/1(WP Fly)
  Logical Operator/1 -> IC1/1
  Subsystem/1(Just Enab) -> Transition/1
